simulink model "MRAC"  (R2022a)
settings: Solver=FixedStepAuto  StartTime=0.0  StopTime=10  FixedStep=0.001  RelTol=1e-3
settings Model: Creator=benja  LastModifiedBy=benja

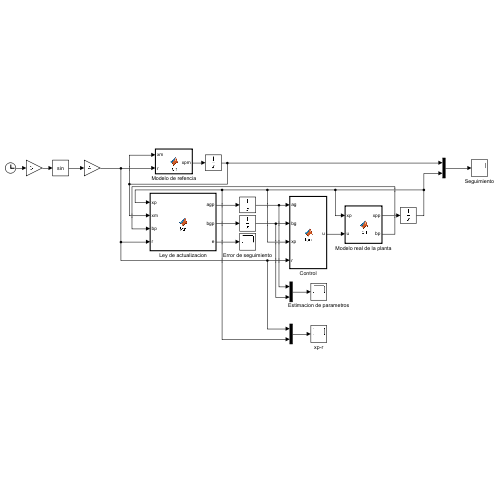
[thumbnail: Simulink's stored preview of the top-level diagram]
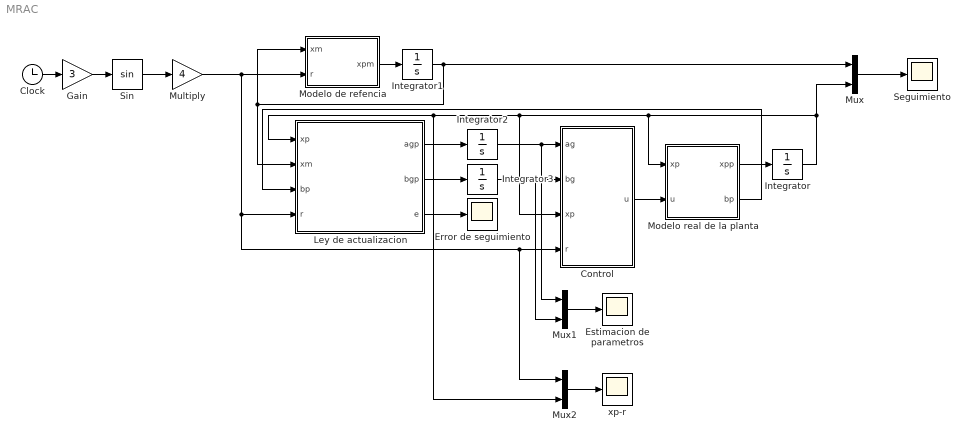
== system MRAC ==
  Clock : Clock
  Control : MATLAB Function  TreatAsAtomicUnit=on
  Error de seguimiento : Scope
  Estimacion de parametros : Scope
  Gain : Gain  Gain=3
  Integrator{,1..3} (4 alike) : Integrator
  Ley de actualizacion : MATLAB Function  TreatAsAtomicUnit=on
  Modelo de refencia : MATLAB Function  TreatAsAtomicUnit=on
  Modelo real de la planta : MATLAB Function  TreatAsAtomicUnit=on
  Multiply : Gain  Gain=4
  Mux : Mux  Inputs=2
  Mux1 : Mux  Inputs=2
  Mux2 : Mux  Inputs=2
  Seguimiento : Scope
  Sin : Trigonometry
  xp-r : Scope
  wires:
  Modelo real de la planta/1(xpp) -> Integrator/1
  Integrator/1 -> Mux2/2, Ley de actualizacion/1(xp), Control/3(xp), Modelo real de la planta/1(xp), Mux/2
  Modelo de refencia/1(xpm) -> Integrator1/1
  Integrator1/1 -> Mux/1, Modelo de refencia/1(xm), Ley de actualizacion/2(xm)
  Control/1(u) -> Modelo real de la planta/2(u)
  Modelo real de la planta/2(bp) -> Ley de actualizacion/3(bp)
  Ley de actualizacion/1(agp) -> Integrator2/1
  Integrator2/1 -> Control/1(ag), Mux1/1
  Ley de actualizacion/2(bgp) -> Integrator3/1
  Integrator3/1 -> Mux1/2, Control/2(bg)
  Mux/1 -> Seguimiento/1
  Multiply/1 -> Mux2/1, Control/4(r), Ley de actualizacion/4(r), Modelo de refencia/2(r)
  Ley de actualizacion/3(e) -> Error de seguimiento/1
  Mux1/1 -> Estimacion de parametros/1
  Gain/1 -> Sin/1
  Clock/1 -> Gain/1
  Sin/1 -> Multiply/1
  Mux2/1 -> xp-r/1

== matlab function MRAC/Modelo de refencia ==
  data: xm input; xpm output; r input
function xpm = fcn(xm, r)

am = -4;
bm = 4;

xpm = am*xm + bm*r;

== matlab function MRAC/Modelo real de la planta ==
  data: xp input; xpp output; u input; bp output
function [xpp, bp] = fcn(xp, u )
ap = -1 
bp = 3
xpp = ap*xp + bp*u;

== matlab function MRAC/Control ==
  data: ag input; u output; bg input; xp input; r input
function u = fcn(ag, bg, xp, r)

u = ag*xp+bg*r;

== matlab function MRAC/Ley de actualizacion ==
  data: agp output; xp input; xm input; bp input; bgp output; r input; e output
function [agp, bgp, e] = fcn( xp, xm, bp, r)

e = xp - xm

agp = -sign(bp)*e*xp
bgp = -sign(bp)*e*r
